simulink library "SLUGS_Library"  (Simulink 7.8)
settings: Solver=ode45  SolverMode=SingleTasking  StartTime=0.0  StopTime=10.0  RelTol=1e-3
values from neighbouring files (symbols this model uses):
  apSampleTime = 0.01    [mcuInit.m]
  derivativesConstant = 5    [mcuInit.m]
  latlong_WP = 1    [mcuInit.m]
  T = 0.01    [mcuInit.m]
  Xpoints = [0 0]    [mcuInit.m]
  Ypoints = [0 0]    [mcuInit.m]
  Zpoints = [0 0]    [mcuInit.m]
undefined symbols (not defined in the file or in its folder): bankCommandLimit, barAdjust, baroCutTemp, baroOffset, baroScale, barTGain1, barTGain2, barTMean1, barTMean2, baseHeight, baseTemp, daLimit, deLimit, DiscIntNeverNeededParam, drLimit, dtLimit, gaind, getGSLocation, getWP, GS_location, Init_onlyOnce, Init_Reset, IPStar, ISA_g, lapseRate, mass, maxAcc, MaxDwnPthStar, maxDynPressure, maxEta, Ndelay, param, pitAdjust, pitchCommandLimit, pitCutTemp, pitotOffset, pitotScale, pitTGain1, pitTGain2, pitTMean1, pitTMean2, polesd, pressureSensorCutoff, rollControlLimit, SampleT, setDiagnosticFloat, setDiagnosticShort, setLogFloat1, setLogFloat2, setNavLong, setNavNav, tanIntercept, Ts, u1, y1, yawDamperLimit, yo, zerosd
libraries: SLUGS_Library x90, simulink x37, dsPICdrivers x33, aerolibconvert2 x4, aerolibutil x1, aerolibobsolete x1
(part 6 of 7)

== system SLUGS_Library/Control Blocks/Control Blocks Examples/PID Controller w/Anti-Windup/Trapezoidal Integrator/Protect NaNs  ==
  In1 : Inport
  Integer Delay3 : Delay  DelayLength=1  InputProcessing=Inherited  SampleTime=T
  Relational Operator2 : RelationalOperator  Operator===  OutDataTypeStr=uint(8)
  Switch3 : Switch  Criteria=u2 > Threshold  Threshold=0.3  SampleTime=.01
  Out1 : Outport
  wires:
  Integer Delay3/1 -> Switch3/3
  Switch3/1 -> Out1/1, Integer Delay3/1
  In1/1 -> Relational Operator2/2, Relational Operator2/1, Switch3/1
  Relational Operator2/1 -> Switch3/2

== system SLUGS_Library/Control Blocks/Control Blocks Examples/PID Controller w/Anti-Windup/Trapezoidal Integrator/Protect NaNs1 ==
  In1 : Inport
  Integer Delay3 : Delay  DelayLength=1  InputProcessing=Inherited  SampleTime=T
  Relational Operator2 : RelationalOperator  Operator===  OutDataTypeStr=uint(8)
  Switch3 : Switch  Criteria=u2 > Threshold  Threshold=0.3  SampleTime=.01
  Out1 : Outport
  wires:
  Integer Delay3/1 -> Switch3/3
  Switch3/1 -> Out1/1, Integer Delay3/1
  In1/1 -> Relational Operator2/2, Relational Operator2/1, Switch3/1
  Relational Operator2/1 -> Switch3/2

== system SLUGS_Library/Control Blocks/Lateral Channel/Roll Control [PID]/Trapezoidal Integrator/Protect NaNs  ==
  In1 : Inport
  Integer Delay3 : Delay  DelayLength=1  InputProcessing=Inherited  SampleTime=T
  Relational Operator2 : RelationalOperator  Operator===  OutDataTypeStr=uint(8)
  Switch3 : Switch  Criteria=u2 > Threshold  Threshold=0.3  SampleTime=.01
  Out1 : Outport
  wires:
  Relational Operator2/1 -> Switch3/2
  In1/1 -> Switch3/1, Relational Operator2/1, Relational Operator2/2
  Switch3/1 -> Integer Delay3/1, Out1/1
  Integer Delay3/1 -> Switch3/3

== system SLUGS_Library/Control Blocks/Lateral Channel/Roll Control [PID]/Trapezoidal Integrator/Protect NaNs1 ==
  In1 : Inport
  Integer Delay3 : Delay  DelayLength=1  InputProcessing=Inherited  SampleTime=T
  Relational Operator2 : RelationalOperator  Operator===  OutDataTypeStr=uint(8)
  Switch3 : Switch  Criteria=u2 > Threshold  Threshold=0.3  SampleTime=.01
  Out1 : Outport
  wires:
  Relational Operator2/1 -> Switch3/2
  In1/1 -> Switch3/1, Relational Operator2/1, Relational Operator2/2
  Switch3/1 -> Integer Delay3/1, Out1/1
  Integer Delay3/1 -> Switch3/3

== system SLUGS_Library/Control Blocks/Lateral Channel/Sideslip Compensation/Low Pass/Compute Coef ==
  a : Inport
  Enable : EnablePort
  -T : Gain  Gain=-apSampleTime  SampleTime=apSampleTime
  1-c : Sum  Inputs=-+  OutDataTypeStr=single  SampleTime=apSampleTime
  Constant : Constant
  Math Function : Math  SaturateOnIntegerOverflow=on
  b : Outport
  c : Outport  Port=2
  wires:
  a/1 -> -T/1
  1-c/1 -> b/1
  Constant/1 -> 1-c/2
  Math Function/1 -> c/1, 1-c/1  "c"
  -T/1 -> Math Function/1

== system SLUGS_Library/Control Blocks/Lateral Channel/Sideslip Compensation/Low Pass/Detect Change ==
  Data : Inport
  Abs1 : Abs  SampleTime=apSampleTime
  Difference1 : simulink/Discrete/Difference  ICPrevInput=0.0  InputProcessing=Inherited  OutMin=[]  OutMax=[]  OutDataType=sfix(16)  OutScaling=2^-10  DoSatur=off
  Saturation1 : Saturate  UpperLimit=1  LowerLimit=0  SampleTime=apSampleTime
  change? : Outport
  wires:
  Saturation1/1 -> change?/1
  Data/1 -> Difference1/1
  Abs1/1 -> Saturation1/1
  Difference1/1 -> Abs1/1

== system SLUGS_Library/Control Blocks/Lateral Channel/Yaw Damper [PID]/Trapezoidal Integrator/Protect NaNs  ==
  In1 : Inport
  Integer Delay3 : Delay  DelayLength=1  InputProcessing=Inherited  SampleTime=T
  Relational Operator2 : RelationalOperator  Operator===  OutDataTypeStr=uint(8)
  Switch3 : Switch  Criteria=u2 > Threshold  Threshold=0.3  SampleTime=.01
  Out1 : Outport
  wires:
  Relational Operator2/1 -> Switch3/2
  In1/1 -> Switch3/1, Relational Operator2/1, Relational Operator2/2
  Switch3/1 -> Integer Delay3/1, Out1/1
  Integer Delay3/1 -> Switch3/3

== system SLUGS_Library/Control Blocks/Lateral Channel/Yaw Damper [PID]/Trapezoidal Integrator/Protect NaNs1 ==
  In1 : Inport
  Integer Delay3 : Delay  DelayLength=1  InputProcessing=Inherited  SampleTime=T
  Relational Operator2 : RelationalOperator  Operator===  OutDataTypeStr=uint(8)
  Switch3 : Switch  Criteria=u2 > Threshold  Threshold=0.3  SampleTime=.01
  Out1 : Outport
  wires:
  Relational Operator2/1 -> Switch3/2
  In1/1 -> Switch3/1, Relational Operator2/1, Relational Operator2/2
  Switch3/1 -> Integer Delay3/1, Out1/1
  Integer Delay3/1 -> Switch3/3

== system SLUGS_Library/Control Blocks/Longitudinal Channel/Airspeed Hold [PID]/Trapezoidal Integrator/Protect NaNs  ==
  In1 : Inport
  Integer Delay3 : Delay  DelayLength=1  InputProcessing=Inherited  SampleTime=T
  Relational Operator2 : RelationalOperator  Operator===  OutDataTypeStr=uint(8)
  Switch3 : Switch  Criteria=u2 > Threshold  Threshold=0.3  SampleTime=.01
  Out1 : Outport
  wires:
  Relational Operator2/1 -> Switch3/2
  In1/1 -> Switch3/1, Relational Operator2/1, Relational Operator2/2
  Switch3/1 -> Integer Delay3/1, Out1/1
  Integer Delay3/1 -> Switch3/3

== system SLUGS_Library/Control Blocks/Longitudinal Channel/Airspeed Hold [PID]/Trapezoidal Integrator/Protect NaNs1 ==
  In1 : Inport
  Integer Delay3 : Delay  DelayLength=1  InputProcessing=Inherited  SampleTime=T
  Relational Operator2 : RelationalOperator  Operator===  OutDataTypeStr=uint(8)
  Switch3 : Switch  Criteria=u2 > Threshold  Threshold=0.3  SampleTime=.01
  Out1 : Outport
  wires:
  Relational Operator2/1 -> Switch3/2
  In1/1 -> Switch3/1, Relational Operator2/1, Relational Operator2/2
  Switch3/1 -> Integer Delay3/1, Out1/1
  Integer Delay3/1 -> Switch3/3

== system SLUGS_Library/Control Blocks/Longitudinal Channel/Height Error to Pitch  Command [PI]/Trapezoidal Integrator/Protect NaNs ==
  In1 : Inport
  Integer Delay3 : Delay  DelayLength=1  InputProcessing=Inherited  SampleTime=T
  Relational Operator2 : RelationalOperator  Operator===  OutDataTypeStr=uint(8)
  Switch3 : Switch  Criteria=u2 > Threshold  Threshold=0.3  SampleTime=.01
  Out1 : Outport
  wires:
  Relational Operator2/1 -> Switch3/2
  In1/1 -> Switch3/1, Relational Operator2/1, Relational Operator2/2
  Switch3/1 -> Integer Delay3/1, Out1/1
  Integer Delay3/1 -> Switch3/3

== system SLUGS_Library/Control Blocks/Longitudinal Channel/Height Error to Pitch  Command [PI]/Trapezoidal Integrator/Protect NaNs  ==
  In1 : Inport
  Integer Delay3 : Delay  DelayLength=1  InputProcessing=Inherited  SampleTime=T
  Relational Operator2 : RelationalOperator  Operator===  OutDataTypeStr=uint(8)
  Switch3 : Switch  Criteria=u2 > Threshold  Threshold=0.3  SampleTime=.01
  Out1 : Outport
  wires:
  Relational Operator2/1 -> Switch3/2
  In1/1 -> Switch3/1, Relational Operator2/1, Relational Operator2/2
  Switch3/1 -> Integer Delay3/1, Out1/1
  Integer Delay3/1 -> Switch3/3

== system SLUGS_Library/Control Blocks/Longitudinal Channel/Pitch To Elevator [PID]/Trapezoidal Integrator/Protect NaNs  ==
  In1 : Inport
  Integer Delay3 : Delay  DelayLength=1  InputProcessing=Inherited  SampleTime=T
  Relational Operator2 : RelationalOperator  Operator===  OutDataTypeStr=uint(8)
  Switch3 : Switch  Criteria=u2 > Threshold  Threshold=0.3  SampleTime=.01
  Out1 : Outport
  wires:
  Relational Operator2/1 -> Switch3/2
  In1/1 -> Switch3/1, Relational Operator2/1, Relational Operator2/2
  Switch3/1 -> Integer Delay3/1, Out1/1
  Integer Delay3/1 -> Switch3/3

== system SLUGS_Library/Control Blocks/Longitudinal Channel/Pitch To Elevator [PID]/Trapezoidal Integrator/Protect NaNs1 ==
  In1 : Inport
  Integer Delay3 : Delay  DelayLength=1  InputProcessing=Inherited  SampleTime=T
  Relational Operator2 : RelationalOperator  Operator===  OutDataTypeStr=uint(8)
  Switch3 : Switch  Criteria=u2 > Threshold  Threshold=0.3  SampleTime=.01
  Out1 : Outport
  wires:
  Relational Operator2/1 -> Switch3/2
  In1/1 -> Switch3/1, Relational Operator2/1, Relational Operator2/2
  Switch3/1 -> Integer Delay3/1, Out1/1
  Integer Delay3/1 -> Switch3/3

== system SLUGS_Library/InnerLoop/Longitudinal Channel/Airspeed Hold [PID]/Trapezoidal Integrator/Protect NaNs  ==
  In1 : Inport
  Integer Delay3 : Delay  DelayLength=1  InputProcessing=Inherited  SampleTime=T
  Relational Operator2 : RelationalOperator  Operator===  OutDataTypeStr=uint(8)
  Switch3 : Switch  Criteria=u2 > Threshold  Threshold=0.3  SampleTime=.01
  Out1 : Outport
  wires:
  Integer Delay3/1 -> Switch3/3
  Switch3/1 -> Out1/1, Integer Delay3/1
  In1/1 -> Relational Operator2/2, Relational Operator2/1, Switch3/1
  Relational Operator2/1 -> Switch3/2

== system SLUGS_Library/InnerLoop/Longitudinal Channel/Airspeed Hold [PID]/Trapezoidal Integrator/Protect NaNs1 ==
  In1 : Inport
  Integer Delay3 : Delay  DelayLength=1  InputProcessing=Inherited  SampleTime=T
  Relational Operator2 : RelationalOperator  Operator===  OutDataTypeStr=uint(8)
  Switch3 : Switch  Criteria=u2 > Threshold  Threshold=0.3  SampleTime=.01
  Out1 : Outport
  wires:
  Integer Delay3/1 -> Switch3/3
  Switch3/1 -> Out1/1, Integer Delay3/1
  In1/1 -> Relational Operator2/2, Relational Operator2/1, Switch3/1
  Relational Operator2/1 -> Switch3/2

== system SLUGS_Library/InnerLoop/Longitudinal Channel/Height Error to Pitch  Command [PI]/Trapezoidal Integrator/Protect NaNs ==
  In1 : Inport
  Integer Delay3 : Delay  DelayLength=1  InputProcessing=Inherited  SampleTime=T
  Relational Operator2 : RelationalOperator  Operator===  OutDataTypeStr=uint(8)
  Switch3 : Switch  Criteria=u2 > Threshold  Threshold=0.3  SampleTime=.01
  Out1 : Outport
  wires:
  Integer Delay3/1 -> Switch3/3
  Switch3/1 -> Out1/1, Integer Delay3/1
  In1/1 -> Relational Operator2/2, Relational Operator2/1, Switch3/1
  Relational Operator2/1 -> Switch3/2

== system SLUGS_Library/InnerLoop/Longitudinal Channel/Height Error to Pitch  Command [PI]/Trapezoidal Integrator/Protect NaNs  ==
  In1 : Inport
  Integer Delay3 : Delay  DelayLength=1  InputProcessing=Inherited  SampleTime=T
  Relational Operator2 : RelationalOperator  Operator===  OutDataTypeStr=uint(8)
  Switch3 : Switch  Criteria=u2 > Threshold  Threshold=0.3  SampleTime=.01
  Out1 : Outport
  wires:
  Integer Delay3/1 -> Switch3/3
  Switch3/1 -> Out1/1, Integer Delay3/1
  In1/1 -> Relational Operator2/2, Relational Operator2/1, Switch3/1
  Relational Operator2/1 -> Switch3/2

== system SLUGS_Library/InnerLoop/Longitudinal Channel/Pitch To Elevator [PID]/Trapezoidal Integrator/Protect NaNs  ==
  In1 : Inport
  Integer Delay3 : Delay  DelayLength=1  InputProcessing=Inherited  SampleTime=T
  Relational Operator2 : RelationalOperator  Operator===  OutDataTypeStr=uint(8)
  Switch3 : Switch  Criteria=u2 > Threshold  Threshold=0.3  SampleTime=.01
  Out1 : Outport
  wires:
  Integer Delay3/1 -> Switch3/3
  Switch3/1 -> Out1/1, Integer Delay3/1
  In1/1 -> Relational Operator2/2, Relational Operator2/1, Switch3/1
  Relational Operator2/1 -> Switch3/2

== system SLUGS_Library/InnerLoop/Longitudinal Channel/Pitch To Elevator [PID]/Trapezoidal Integrator/Protect NaNs1 ==
  In1 : Inport
  Integer Delay3 : Delay  DelayLength=1  InputProcessing=Inherited  SampleTime=T
  Relational Operator2 : RelationalOperator  Operator===  OutDataTypeStr=uint(8)
  Switch3 : Switch  Criteria=u2 > Threshold  Threshold=0.3  SampleTime=.01
  Out1 : Outport
  wires:
  Integer Delay3/1 -> Switch3/3
  Switch3/1 -> Out1/1, Integer Delay3/1
  In1/1 -> Relational Operator2/2, Relational Operator2/1, Switch3/1
  Relational Operator2/1 -> Switch3/2

== system SLUGS_Library/InnerLoop/Navigation/Compute WP Index/Compute Modified L1/Compute T  in Frenet ==
  Pos 1 : Inport
  Pos 2 : Inport  Port=2
  Add : Sum  Inputs=-+
  Normalize Vector : SLUGS_Library/Navigation/Normalize Vector
  T : Outport
  wires:
  Pos 1/1 -> Add/1
  Pos 2/1 -> Add/2
  Add/1 -> Normalize Vector/1
  Normalize Vector/1 -> T/1

== system SLUGS_Library/InnerLoop/Navigation/Compute WP Index/Compute Modified L1/Get Circles ==
  T1 : Inport
  T2 : Inport  Port=2
  "Wp_to " : Inport  Port=3
  R : Inport  Port=4
  Compute  Circles : MATLAB Function  TreatAsAtomicUnit=on
  Compute CCW Angle From 2 Vectors : Subsystem
  Compute delta Left Turn : Subsystem
  Constant5 : Constant  Value=pi  OutDataTypeStr=single
  Larger than 180? : RelationalOperator  OutDataTypeStr=boolean
  Logical Operator : Logic  Operator=NOT  AllPortsSameDT=off  OutDataTypeStr=boolean
  Merge4 : Merge
  Subsystem5 : SLUGS_Library/Subsystem5
  To Workspace : ToWorkspace  VariableName=O  SampleTime=-1  SaveFormat=Structure
  To Workspace1 : ToWorkspace  VariableName=P  SampleTime=-1  SaveFormat=Structure
  To Workspace2 : ToWorkspace  VariableName=Pch  SampleTime=-1  SaveFormat=Structure
  To Workspace3 : ToWorkspace  VariableName=PchB  SampleTime=-1  SaveFormat=Structure
  compute delta Right Turn : Subsystem
  P : Outport
  wires:
  Subsystem5/2 -> Compute  Circles/2(cd)
  Subsystem5/1 -> Compute  Circles/1(sd)
  Logical Operator/1 -> Compute delta Left Turn/Enable
  Larger than 180?/1 -> Logical Operator/1, compute delta Right Turn/Enable
  Constant5/1 -> Larger than 180?/2
  Compute  Circles/4(PchB) -> To Workspace3/1
  Compute  Circles/3(Pch) -> To Workspace2/1
  Compute  Circles/2(P) -> To Workspace1/1, P/1
  Compute  Circles/1(O) -> To Workspace/1
  "Wp_to "/1 -> Compute  Circles/3(WP1)
  R/1 -> Compute  Circles/4(R)
  Compute delta Left Turn/1(delta) -> Merge4/2
  compute delta Right Turn/1(delta) -> Merge4/1
  Merge4/1 -> Subsystem5/1
  T2/1 -> Compute CCW Angle From 2 Vectors/2(V), Compute  Circles/6(T2)
  Compute CCW Angle From 2 Vectors/1(CCW Ang) -> Larger than 180?/1, compute delta Right Turn/1(gamma), Compute delta Left Turn/1(gamma)  "gamma"
  T1/1 -> Compute CCW Angle From 2 Vectors/1(U), Compute  Circles/5(T1)

== system SLUGS_Library/InnerLoop/Navigation/Compute WP Index/Compute Modified L1/get WP Coord from Index ==
  WP Idx : Inport
  C Function Call : dsPICdrivers/OTHERS/C Function Call  Tag=dsPIC_dsPIC_CFunctionCall  FctUpdate=Output Function  fctName='getWP'  INPUT_SIZE=1  INPUT1=uint8  INPUT2=--  INPUT3=--  OUTPUT_SIZE=3  OUTPUT1=real32  SampleTime=-1  InputType=[ 2 ]  OutputType=[ 7 ]  FctDeclaration=extern void getWP(uint8_T u1,real32_T* y1);  FctCall=getWP(%u1, *%y1);  OrderingInOutPopup=None  FctStart=None  FctStart_Name=Init_onlyOnce  FctStart_Declaration=inline extern void Init_onlyOnce();  FctStart_Call=Init_onlyOnce();  FctInit=None  FctInit_Name=Init_Reset  FctInit_Declaration=inline extern void Init_Reset();  FctInit_Call=Init_Reset();  PinDigitalInput=[]  PinDigitalOutput=[]  AnalogueInput=[]
  Data Type Conversion : DataTypeConversion  OutDataTypeStr=double
  Data Type Conversion1 : DataTypeConversion  OutDataTypeStr=single
  Environment Controller : simulink/Signal Routing/Environment Controller
  MATLAB Fcn : MATLABFcn  MATLABFcn=Xpoints(u(1))  OutputDimensions=1  OutputSignalType=real
  MATLAB Fcn1 : MATLABFcn  MATLABFcn=Ypoints(u(1))  OutputDimensions=1
  MATLAB Fcn2 : MATLABFcn  MATLABFcn=Zpoints(u(1))  OutputDimensions=1
  Mux : Mux  Inputs=3
  WP Coord : Outport
  wires:
  C Function Call/1 -> Environment Controller/2
  Environment Controller/1 -> WP Coord/1
  Mux/1 -> Data Type Conversion1/1
  WP Idx/1 -> C Function Call/1, Data Type Conversion/1
  MATLAB Fcn2/1 -> Mux/3
  MATLAB Fcn1/1 -> Mux/2
  MATLAB Fcn/1 -> Mux/1
  Data Type Conversion/1 -> MATLAB Fcn1/1, MATLAB Fcn/1, MATLAB Fcn2/1
  Data Type Conversion1/1 -> Environment Controller/1

== system SLUGS_Library/Navigation/Compute WP Index/Compute Modified L1/Get Circles/Compute CCW Angle From 2 Vectors ==
  U : Inport
  V : Inport  Port=2
  Add : Sum  Inputs=+-
  Embedded MATLAB Function1 : MATLAB Function  TreatAsAtomicUnit=on
  Selector : Selector  InputPortWidth=3  IndexOptions=Index vector (dialog)  Indices=[1]  OutputSizes=1
  Selector1 : Selector  InputPortWidth=3  IndexOptions=Index vector (dialog)  Indices=[1]  OutputSizes=1
  Selector2 : Selector  InputPortWidth=3  IndexOptions=Index vector (dialog)  Indices=[2]  OutputSizes=1
  Selector3 : Selector  InputPortWidth=3  IndexOptions=Index vector (dialog)  Indices=[2]  OutputSizes=1
  Subsystem1 : SLUGS_Library/Subsystem4
  Subsystem4 : SLUGS_Library/Subsystem4
  CCW Ang : Outport
  wires:
  Selector3/1 -> Subsystem4/1
  Selector/1 -> Subsystem4/2
  Selector2/1 -> Subsystem1/1
  Selector1/1 -> Subsystem1/2
  Subsystem4/1 -> Add/1
  Subsystem1/1 -> Add/2
  Add/1 -> Embedded MATLAB Function1/1(rawAngle)
  U/1 -> Selector3/1, Selector/1
  V/1 -> Selector2/1, Selector1/1
  Embedded MATLAB Function1/1(angle) -> CCW Ang/1

== system SLUGS_Library/Navigation/Compute WP Index/Compute Modified L1/Get Circles/Compute delta Left Turn ==
  gamma : Inport
  Enable : EnablePort
  Add : Sum  Inputs=+-
  Constant1 : Constant  Value=2
  Constant5 : Constant  Value=pi
  Divide : Product  Inputs=*/
  Gain : Gain  Gain=-1
  delta : Outport
  wires:
  Constant1/1 -> Divide/2
  Divide/1 -> Gain/1
  Constant5/1 -> Add/1
  gamma/1 -> Add/2
  Add/1 -> Divide/1
  Gain/1 -> delta/1

== system SLUGS_Library/Navigation/Compute WP Index/Compute Modified L1/Get Circles/compute delta Right Turn ==
  gamma : Inport
  Enable : EnablePort
  Add : Sum  Inputs=-+
  Constant1 : Constant  Value=2
  Constant5 : Constant  Value=pi
  Divide : Product  Inputs=*/
  delta : Outport
  wires:
  Constant5/1 -> Add/1
  Add/1 -> Divide/1
  Constant1/1 -> Divide/2
  gamma/1 -> Add/2
  Divide/1 -> delta/1  "delta"

== system SLUGS_Library/Navigation/Geod2LTP/ECEF2LTP (UEN)/From Body to Universal1/Rotation Matrix from Long//Lat ==
  note: Calculate Coefficients of DCM Row-Wise
  long lat : Inport
  11 : Fcn  Expr=cos(u[1])*cos(u[2])
  12 : Fcn  Expr=sin(u[1])*cos(u[2])
  13 : Fcn  Expr=sin(u[2])
  21 : Fcn  Expr=-sin(u[1])
  22 : Fcn  Expr=cos(u[1])
  23 : Fcn  Expr=0
  31 : Fcn  Expr=-sin(u[2])*cos(u[1])
  32 : Fcn  Expr=-sin(u[1])*sin(u[2])
  33 : Fcn  Expr=cos(u[2])
  Mux2 : Mux  Inputs=9
  DCM : Outport
  wires:
  long lat/1 -> 21/1, 31/1, 12/1, 22/1, 32/1, 13/1, 23/1, 33/1, 11/1
  Mux2/1 -> DCM/1
  11/1 -> Mux2/1
  21/1 -> Mux2/2
  31/1 -> Mux2/3
  12/1 -> Mux2/4
  22/1 -> Mux2/5
  32/1 -> Mux2/6
  13/1 -> Mux2/7
  23/1 -> Mux2/8
  33/1 -> Mux2/9

== system SLUGS_Library/Navigation/Navigation/L2+/Get Sin, Cos eta/2D Dot Product  ==
  Vxyz : Inport
  L2_vec : Inport  Port=2
  Demux : Demux  Outputs=3
  Demux1 : Demux  Outputs=3
  Product : Product  RndMeth=Zero
  Product1 : Product  RndMeth=Zero
  Subtract : Sum  Inputs=2
  Terminator : Terminator
  Terminator1 : Terminator
  2D _dot : Outport
  wires:
  Vxyz/1 -> Demux/1
  Subtract/1 -> 2D _dot/1
  L2_vec/1 -> Demux1/1
  Product1/1 -> Subtract/2
  Product/1 -> Subtract/1
  Demux1/3 -> Terminator1/1
  Demux/3 -> Terminator/1
  Demux1/1 -> Product/1
  Demux/1 -> Product/2
  Demux1/2 -> Product1/1
  Demux/2 -> Product1/2

== system SLUGS_Library/Navigation/Navigation/L2+/Get Sin, Cos eta/Get  Groundspeed ==
  L2_vec : Inport  SampleTime=apSampleTime
  Vector Norm : SLUGS_Library/Vector Norm
  Zero out Z1 : MATLAB Function  TreatAsAtomicUnit=on
  |L2| : Outport
  wires:
  L2_vec/1 -> Zero out Z1/1(Pin)
  Zero out Z1/1(P) -> Vector Norm/1
  Vector Norm/1 -> |L2|/1

== system SLUGS_Library/Navigation/Navigation/L2+/Get Sin, Cos eta/Get ZProd ==
  L2_vec : Inport
  Vxyz : Inport  Port=2
  Demux : Demux  Outputs=3
  Demux1 : Demux  Outputs=3
  Product : Product  RndMeth=Zero
  Product1 : Product  RndMeth=Zero
  Subtract : Sum  Inputs=+-
  Terminator : Terminator
  Terminator1 : Terminator
  Z_prod : Outport
  wires:
  Demux/3 -> Terminator/1
  Demux1/3 -> Terminator1/1
  Demux/1 -> Product/2
  Demux1/2 -> Product/1
  Demux/2 -> Product1/2
  Demux1/1 -> Product1/1
  Product/1 -> Subtract/1
  Product1/1 -> Subtract/2
  L2_vec/1 -> Demux1/1
  Subtract/1 -> Z_prod/1
  Vxyz/1 -> Demux/1

== system SLUGS_Library/Navigation/Navigation/Normal WP  Navigation/Compute WP Switching Trigger/Compute  Projection ==
  Pned : Inport
  ToWp : Inport  Port=2
  T : Inport  Port=3
  Protect NaNs : Subsystem
  Subtract : Sum  Inputs=-+  OutDataTypeStr=single
  dsPIC Dot Product : SLUGS_Library/dsPIC Dot Product
  D2wp1 : Outport
  wires:
  Protect NaNs/1(Out1) -> D2wp1/1
  Pned/1 -> Subtract/1
  ToWp/1 -> Subtract/2
  Subtract/1 -> dsPIC Dot Product/1
  T/1 -> dsPIC Dot Product/2
  dsPIC Dot Product/1 -> Protect NaNs/1(In1)

== system SLUGS_Library/Navigation/Navigation/Normal WP  Navigation/On WP Enable/Subsystem ==
  GS LLA : Inport
  GS R_in : Inport  Port=2
  Compute Frenet : SLUGS_Library/Navigation/Compute Frenet
  Constant : Constant  OutDataTypeStr=uint8  SampleTime=0.01
  Constant1 : Constant  Value=2  OutDataTypeStr=uint8  SampleTime=0.01
  GS LLA_1 : InportShadow  Port=1
  GS R_in_1 : InportShadow  Port=2
  Terminator : Terminator
  get WP Coord from Index : SLUGS_Library/Navigation/get WP Coord from Index
  get WP Coord from Index1 : SLUGS_Library/Navigation/get WP Coord from Index
  WP0 : Outport
  T1 : Outport  Port=2
  wires:
  GS R_in_1/1 -> get WP Coord from Index1/3
  GS LLA_1/1 -> get WP Coord from Index1/2
  Constant1/1 -> get WP Coord from Index1/1
  get WP Coord from Index1/1 -> Compute Frenet/2
  get WP Coord from Index/1 -> Compute Frenet/1, WP0/1
  GS R_in/1 -> get WP Coord from Index/3
  GS LLA/1 -> get WP Coord from Index/2
  Compute Frenet/1 -> T1/1
  Compute Frenet/2 -> Terminator/1
  Constant/1 -> get WP Coord from Index/1

== system SLUGS_Library/Navigation/Navigation/Recent Enable/Grab Upon Enable/Compute GS Location ==
  GS Location : Inport
  Demux : Demux  Outputs=3
  Geod2ECEF1 : Subsystem  mask{Re=6378137, Rp=6356752.3142}
      mask prompts: Re "Enter equatorial radius, m"; Rp "Enter polar radius,m"
  Mux1 : Mux  Inputs=2
  Mux2 : Mux  Inputs=3
  "Lon, Lat" : Outport
  R_in : Outport  Port=2
  wires:
  Geod2ECEF1/3("Ze, m ") -> Mux2/3
  Geod2ECEF1/1("Xe, m ") -> Mux2/1
  Geod2ECEF1/2("Ye, m ") -> Mux2/2
  Demux/1 -> Geod2ECEF1/1("height, m")
  Demux/2 -> Geod2ECEF1/2("lat, deg"), Mux1/2
  Demux/3 -> Geod2ECEF1/3(lon,deg), Mux1/1
  GS Location/1 -> Demux/1
  Mux1/1 -> "Lon, Lat"/1
  Mux2/1 -> R_in/1  "R_in"

== system SLUGS_Library/Navigation/Navigation/Recent Enable/Subsystem/Detect Rising Edge ==
  In1 : Inport
  Delay : Delay  DelayLength=1
  Logical Operator : Logic  AllPortsSameDT=off  OutDataTypeStr=boolean
  Relational Operator : RelationalOperator  Operator=~=  OutDataTypeStr=boolean
  Out1 : Outport
  wires:
  Logical Operator/1 -> Out1/1
  In1/1 -> Logical Operator/2, Relational Operator/2, Delay/1
  Relational Operator/1 -> Logical Operator/1
  Delay/1 -> Relational Operator/1

== system SLUGS_Library/Sensor Blocks/Baro Alt/Baro Altimeter/Initial Baro Bias/Low Pass8 ==
  In1 : Inport
  Discrete Zero-Pole : DiscreteZeroPole  Zeros=zerosd  Poles=polesd  Gain=gaind  SampleTime=SampleTime
  Out1 : Outport
  wires:
  In1/1 -> Discrete Zero-Pole/1
  Discrete Zero-Pole/1 -> Out1/1

== system SLUGS_Library/InnerLoop/Navigation/Compute WP Index/Compute Modified L1/Get Circles/Compute CCW Angle From 2 Vectors ==
  U : Inport
  V : Inport  Port=2
  Add : Sum  Inputs=+-
  Embedded MATLAB Function1 : MATLAB Function  TreatAsAtomicUnit=on
  Selector : Selector  InputPortWidth=3  IndexOptions=Index vector (dialog)  Indices=[1]  OutputSizes=1
  Selector1 : Selector  InputPortWidth=3  IndexOptions=Index vector (dialog)  Indices=[1]  OutputSizes=1
  Selector2 : Selector  InputPortWidth=3  IndexOptions=Index vector (dialog)  Indices=[2]  OutputSizes=1
  Selector3 : Selector  InputPortWidth=3  IndexOptions=Index vector (dialog)  Indices=[2]  OutputSizes=1
  Subsystem1 : SLUGS_Library/Subsystem4
  Subsystem4 : SLUGS_Library/Subsystem4
  CCW Ang : Outport
  wires:
  Embedded MATLAB Function1/1(angle) -> CCW Ang/1
  V/1 -> Selector1/1, Selector2/1
  U/1 -> Selector/1, Selector3/1
  Add/1 -> Embedded MATLAB Function1/1(rawAngle)
  Subsystem1/1 -> Add/2
  Subsystem4/1 -> Add/1
  Selector1/1 -> Subsystem1/2
  Selector2/1 -> Subsystem1/1
  Selector/1 -> Subsystem4/2
  Selector3/1 -> Subsystem4/1

== system SLUGS_Library/InnerLoop/Navigation/Compute WP Index/Compute Modified L1/Get Circles/Compute delta Left Turn ==
  gamma : Inport
  Enable : EnablePort
  Add : Sum  Inputs=+-  OutDataTypeStr=single
  Constant1 : Constant  Value=2  OutDataTypeStr=single
  Constant5 : Constant  Value=pi  OutDataTypeStr=single
  Divide : Product  Inputs=*/  OutDataTypeStr=single
  Gain : Gain  Gain=-1
  delta : Outport
  wires:
  Gain/1 -> delta/1
  Add/1 -> Divide/1
  gamma/1 -> Add/2
  Constant5/1 -> Add/1
  Divide/1 -> Gain/1
  Constant1/1 -> Divide/2

== system SLUGS_Library/InnerLoop/Navigation/Compute WP Index/Compute Modified L1/Get Circles/compute delta Right Turn ==
  gamma : Inport
  Enable : EnablePort
  Add : Sum  Inputs=-+  OutDataTypeStr=single
  Constant1 : Constant  Value=2  OutDataTypeStr=single
  Constant5 : Constant  Value=pi  OutDataTypeStr=single
  Divide : Product  Inputs=*/  OutDataTypeStr=single
  delta : Outport
  wires:
  Divide/1 -> delta/1  "delta"
  gamma/1 -> Add/2
  Constant1/1 -> Divide/2
  Add/1 -> Divide/1
  Constant5/1 -> Add/1

== system SLUGS_Library/Navigation/Navigation/Normal WP  Navigation/Compute WP Switching Trigger/Compute  Projection/Protect NaNs ==
  In1 : Inport
  Integer Delay3 : Delay  DelayLength=1  InputProcessing=Inherited  SampleTime=T
  Relational Operator2 : RelationalOperator  Operator===  OutDataTypeStr=uint(8)
  Switch3 : Switch  Criteria=u2 > Threshold  Threshold=0.3  SampleTime=.01
  Out1 : Outport
  wires:
  Integer Delay3/1 -> Switch3/3
  Switch3/1 -> Out1/1, Integer Delay3/1
  In1/1 -> Relational Operator2/2, Relational Operator2/1, Switch3/1
  Relational Operator2/1 -> Switch3/2

== system SLUGS_Library/Navigation/Navigation/Recent Enable/Grab Upon Enable/Compute GS Location/Geod2ECEF1 ==
  "height, m" : Inport
  "lat, deg" : Inport  Port=2
  lon,deg : Inport  Port=3
  (Rh+h)cos(phi)*cos(lamb)=Xe : Product  Inputs=3  OutDataTypeStr=single  SaturateOnIntegerOverflow=on  InputSameDT=on
  (Rh+h)cos(phi)*sin(lamb)=Ye : Product  Inputs=3  OutDataTypeStr=single  SaturateOnIntegerOverflow=on  InputSameDT=on
  Deg2R : Gain  Gain=pi/180  OutDataTypeStr=float('single')  SaturateOnIntegerOverflow=on  ParamDataTypeStr=Inherit: Same as input
  Deg2R1 : Gain  Gain=pi/180  OutDataTypeStr=float('single')  SaturateOnIntegerOverflow=on  ParamDataTypeStr=Inherit: Same as input
  Product1 : Product  SaturateOnIntegerOverflow=on  InputSameDT=on  OutDataTypeStr=Inherit: Same as first input
  Re=equatorial radius : Constant  Value=Re  OutDataTypeStr=single
  Rh : Product  Inputs=*/  OutDataTypeStr=single  SaturateOnIntegerOverflow=on  InputSameDT=on
  Rh(1-e^2) : Product  OutDataTypeStr=single  SaturateOnIntegerOverflow=on  InputSameDT=on
  Sum1 : Sum  Inputs=+-|  SaturateOnIntegerOverflow=on  InputSameDT=on  OutDataTypeStr=Inherit: Same as first input
  Sum2 : Sum  SaturateOnIntegerOverflow=on  InputSameDT=on  OutDataTypeStr=Inherit: Same as first input
      settings: AttributesFormatString=Rh+h
  Sum3 : Sum  Inputs=|+-  SaturateOnIntegerOverflow=on  InputSameDT=on  OutDataTypeStr=Inherit: Same as first input
  Sum4 : Sum  OutDataTypeStr=single  SaturateOnIntegerOverflow=on  InputSameDT=on
      settings: AttributesFormatString=(1-e^2)Rh+h
  Ze : Product  OutDataTypeStr=single  SaturateOnIntegerOverflow=on  InputSameDT=on
  const : Constant  OutDataTypeStr=single
  const1 : Constant  OutDataTypeStr=single
  cos(lamb) : Trigonometry  Operator=cos
  cos(phi) : Trigonometry  Operator=cos
  eccentricity^2 : Subsystem
  f : Fcn  Expr=sqrt(u(1))
  sin(lamb) : Trigonometry
  sin(phi) : Trigonometry
  sin(phi)^2 : Product  SaturateOnIntegerOverflow=on  InputSameDT=on  OutDataTypeStr=Inherit: Same as first input
  "Xe, m " : Outport
  "Ye, m " : Outport  Port=2
  "Ze, m " : Outport  Port=3
  wires:
  (Rh+h)cos(phi)*sin(lamb)=Ye/1 -> "Ye, m "/1
  (Rh+h)cos(phi)*cos(lamb)=Xe/1 -> "Xe, m "/1
  Sum2/1 -> (Rh+h)cos(phi)*cos(lamb)=Xe/1, (Rh+h)cos(phi)*sin(lamb)=Ye/1
  Deg2R1/1 -> sin(lamb)/1, cos(lamb)/1
  Deg2R/1 -> sin(phi)/1, cos(phi)/1
  Ze/1 -> "Ze, m "/1
  sin(lamb)/1 -> (Rh+h)cos(phi)*sin(lamb)=Ye/3
  cos(lamb)/1 -> (Rh+h)cos(phi)*cos(lamb)=Xe/3
  cos(phi)/1 -> (Rh+h)cos(phi)*sin(lamb)=Ye/2, (Rh+h)cos(phi)*cos(lamb)=Xe/2
  lon,deg/1 -> Deg2R1/1
  Sum4/1 -> Ze/2
  Rh(1-e^2)/1 -> Sum4/1
  Sum3/1 -> Rh(1-e^2)/1  "1-e^2"
  const1/1 -> Sum3/1
  sin(phi)^2/1 -> Product1/2
  eccentricity^2/1(e^2) -> Sum3/2, Product1/1
  "height, m"/1 -> Sum2/1, Sum4/2
  const/1 -> Sum1/1
  Sum1/1 -> f/1
  Product1/1 -> Sum1/2
  Rh/1 -> Rh(1-e^2)/2, Sum2/2
  Re=equatorial radius/1 -> Rh/1
  f/1 -> Rh/2
  sin(phi)/1 -> Ze/1, sin(phi)^2/2, sin(phi)^2/1
  "lat, deg"/1 -> Deg2R/1

== system SLUGS_Library/Navigation/Navigation/Recent Enable/Grab Upon Enable/Compute GS Location/Geod2ECEF1/eccentricity^2 ==
  " " : Product  OutDataTypeStr=single  SaturateOnIntegerOverflow=on  InputSameDT=on
  Re=equatorial radius1 : Constant  Value=Re  OutDataTypeStr=single
  Rp=polar radius : Constant  Value=Rp  OutDataTypeStr=single
  Sum5 : Sum  Inputs=|+-  SaturateOnIntegerOverflow=on  InputSameDT=on  OutDataTypeStr=Inherit: Same as first input
  const2 : Constant  OutDataTypeStr=single
  e^1 : Product  Inputs=*/  OutDataTypeStr=single  SaturateOnIntegerOverflow=on  InputSameDT=on
  e^2 : Outport
  wires:
  Sum5/1 -> e^2/1
  " "/1 -> Sum5/2
  e^1/1 -> " "/1, " "/2
  const2/1 -> Sum5/1
  Rp=polar radius/1 -> e^1/1
  Re=equatorial radius1/1 -> e^1/2

== matlab function Singnal Routing & Conditioning/3D Filter/myMux Fun1 ==
  data: u1 input double; y output double; u2 input double; u3 input double
function y = myMux(u1, u2, u3)
% This block supports an embeddable subset of the MATLAB language.
% See the help menu for details. 

y = [u1(1); u2(1); u3(1)];

== matlab function Navigation/Compute Frenet/Select N Terms ==
  data: T input double; N output double
function N = getN(T)
% This block supports an embeddable subset of the MATLAB language.
% See the help menu for details. 

N = [-T(2); T(1); 0];

== matlab function Navigation/Compute WP Index/Compute Modified L1/Get Circles/Compute CCW Angle From 2 Vectors/Embedded MATLAB Function1 ==
  data: rawAngle input double; angle output double
function angle = mapToTwoPi(rawAngle)

 if(rawAngle < 0)
  angle = rawAngle + 2*pi;
 else
  angle = rawAngle;   
 end

== matlab function Compute CCW Angle From 2 Vectors/Embedded MATLAB Function1 ==
  data: rawAngle input double; angle output double
function angle = mapToTwoPi(rawAngle)

angle = rawAngle;

 if(angle < 0)
     while (angle <0)
        angle = angle + 2*pi;
     end;
 else
     while (angle > 2*pi)
        angle = angle - 2*pi;
     end
 end

== matlab function dsPIC Dot Product/Embedded MATLAB Function ==
  data: x input double; y input double; xDoty output double
function xDoty = myDot(x,y)
% This block supports an embeddable subset of the MATLAB language.
% See the help menu for details. 

xDoty = x(1)*y(1) + x(2)*y(2) + x(3)*y(3);

== matlab function Embedded MATLAB Function ==
  data: T1 input double; gamma output double; T2 input double
function gamma = computeAngle(T1, T2)
% This block supports an embeddable subset of the MATLAB language.
% See the help menu for details. 

gamma = (atan2(T1(2), T1(1)) - atan2(T2(2), T2(1)));

 if(gamma < 0)
  gamma = gamma + 2*pi;
 end

== matlab function Navigation/Compute WP Index/Embedded MATLAB Function ==
  data: wpStart input double; wpCount input double; wp0 output double; swIncrement input double; wp1 output double; wp2 output double; wpEnabl input double
function [wp0,wp1, wp2] = getNextWP(wpStart, wpCount, swIncrement, wpEnabl)

% Declare static variables
persistent fromWP;
persistent toWP;
persistent totoWP;

%initialize the static variables
if isempty(fromWP)
    fromWP = wpStart;
    toWP = fromWP+1;
    % check if there are more than 2 WPs
    if wpCount > toWP + 1
        totoWP = toWP+1;
    else
        totoWP = fromWP;
    end
end

%if WP Nav was just enabled
if wpEnabl == 1
    fromWP =0;
    toWP =1;
    totoWP = 2;
end;

% if there is a change of wp
if swIncrement == 1
    fromWP = toWP;
    toWP = totoWP;
    totoWP = totoWP +1;
    if (totoWP>wpCount)
        totoWP = wpStart;
    end
end

wp0 = fromWP;
wp1 = toWP;
wp2 = totoWP;

== matlab function InnerLoop/Navigation/Compute WP Index/Compute Modified L1/Get Circles/Compute Circles ==
  data: sd input double; O output double; cd input double; WP1 input double; R input double; T1 input double; P output double; Pch output double; T2 input double; PchB output double
function [O,P,Pch, PchB] = getO(sd, cd, WP1, R, T1, T2)
    % This block supports an embeddable subset of the MATLAB language.
    % See the help menu for details.

    % rotate the vector delta degrees
    r_vec = zeros(3,1);
    r_vec(1) = -T1(1)*cd -T1(2)*sd;
    r_vec(2) = T1(1)*sd -T1(2)*cd;

    %compute M
    if localAbs(sd)>0.01
        M = localAbs(R/sd);
    else
        M = single(0);
    end

    %find the distance from WP
    P = M*cd;

    % find the center of the circle
    O = WP1 + r_vec.*M;

    % find the tangent points
    Pch = WP1-T1*P;
    PchB = WP1 + T2*P;
end

function absVal = localAbs(x)
    if x < 0
        absVal = single(-1*x);
    else
        absVal = single(x);
    end
end

== matlab function InnerLoop/Navigation/Compute WP Index/Compute Modified L1/Get Circles/Compute CCW Angle From 2 Vectors/Embedded MATLAB Function1 ==
  data: rawAngle input double; angle output double
function angle = mapToTwoPi(rawAngle)

 if(rawAngle < 0)
  angle = rawAngle + 2*pi;
 else
  angle = rawAngle;   
 end

== matlab function InnerLoop/Navigation/Compute WP Index/Embedded MATLAB Function ==
  data: wpStart input double; wpCount input double; wp0 output double; swIncrement input double; wp1 output double; wp2 output double; wpEnabl input double
function [wp0,wp1, wp2] = getNextWP(wpStart, wpCount, swIncrement, wpEnabl)

% Declare static variables
persistent fromWP;
persistent toWP;
persistent totoWP;

%initialize the static variables
if isempty(fromWP)
    fromWP = uint8(wpStart);
    toWP = uint8(fromWP+1);
    % check if there are more than 2 WPs
    if wpCount > toWP + 1
        totoWP = uint8(toWP+1);
    else
        totoWP = uint8(fromWP);
    end
end

%if WP Nav was just enabled
if wpEnabl == 1
    fromWP = uint8(0);
    toWP = uint8(1);
    totoWP = uint8(2);
end;

% if there is a change of wp
if swIncrement == 1
    fromWP = toWP;
    toWP = totoWP;
    totoWP = totoWP +1;
    if (totoWP>wpCount)
        totoWP = wpStart;
    end
end

wp0 = fromWP;
wp1 = toWP;
wp2 = totoWP;

== matlab function negprotect ==
  data: val input double; zpVal output double
function zpVal = negProt(val)
% This block supports an embeddable subset of the MATLAB language.
% See the help menu for details. 

if val >= single(0.001)
    zpVal = val;
else
    zpVal = single(0.001);
end

== matlab function Navigation/Compute WP Index/Compute Modified L1/Get Circles/Compute Circles ==
  data: sd input double; O output double; cd input double; WP1 input double; R input double; T1 input double; P output double; Pch output double; T2 input double; PchB output double
function [O,P,Pch, PchB] = getO(sd, cd, WP1, R, T1, T2)
    % This block supports an embeddable subset of the MATLAB language.
    % See the help menu for details.

    % rotate the vector delta degrees
    r_vec = zeros(3,1);
    r_vec(1) = -T1(1)*cd -T1(2)*sd;
    r_vec(2) = T1(1)*sd -T1(2)*cd;

    %compute M
    if localAbs(sd)>0.01
        M = localAbs(R/sd);
    else
        M = 0;
    end

    %find the distance from WP
    P = M*cd;

    % find the center of the circle
    O = WP1 + r_vec.*M;

    % find the tangent points
    Pch = WP1-T1*P;
    PchB = WP1 + T2*P;
end

function absVal = localAbs(x)
    if x < 0
        absVal = -1*x;
    else
        absVal = x;
    end
end

== matlab function dsPIC_SQRT/negprotect ==
  data: val input double; zpVal output double
function zpVal = negProt(val)
% This block supports an embeddable subset of the MATLAB language.
% See the help menu for details. 

if val >= single(0.001)
    zpVal = val;
else
    zpVal = single(0.001);
end

== matlab function Navigation/Bank to Psi Dot/negprotect ==
  data: val input double; zpVal output double
function zpVal = negProt(val)
% This block supports an embeddable subset of the MATLAB language.
% See the help menu for details. 

if val >= single(0.001)
    zpVal = val;
else
    zpVal = single(0.001);
end

== matlab function Navigation/Park, Deyst & How Lat Accel Cmd/Compute Eta/negprotect ==
  data: val input double; zpVal output double
function zpVal = negProt(val)
% This block supports an embeddable subset of the MATLAB language.
% See the help menu for details. 

if val >= single(0.001)
    zpVal = val;
else
    zpVal = single(0.001);
end

== matlab function Navigation/Park, Deyst & How Lat Accel Cmd/Compute Eta/negprotect1 ==
  data: val input double; zpVal output double
function zpVal = negProt(val)
% This block supports an embeddable subset of the MATLAB language.
% See the help menu for details. 

if val >= single(0.001)
    zpVal = val;
else
    zpVal = single(0.001);
end

== matlab function Singnal Routing & Conditioning/myMux Fun3 ==
  data: u1 input double; y output double; u2 input double; u3 input double
function y = myMux(u1, u2, u3)
% This block supports an embeddable subset of the MATLAB language.
% See the help menu for details. 

y = [u1(1); u2(1); u3(1)];

== matlab function Singnal Routing & Conditioning/3D LowPass w/Initial Condition/myMux Fun1 ==
  data: u1 input double; y output double; u2 input double; u3 input double
function y = myMux(u1, u2, u3)
% This block supports an embeddable subset of the MATLAB language.
% See the help menu for details. 

y = [u1(1); u2(1); u3(1)];

== matlab function InnerLoop/Longitudinal Channel/0.5 sec  tau for Turns/Embedded MATLAB Function ==
  data: u input double; y output double; T input double; f input double
function y = fcn(u,T,f)
% This block supports an embeddable subset of the MATLAB language.
% See the help menu for details. 

persistent a
persistent b
persistent y_km1
persistent u_km1
if isempty(a)
    %tf = [T*omega/(2+T*omega) T*omega/(2+T*omega)],[1 (T*omega-2)/(T*omega+2)]
    %tf = [a a],[1 -b]
    omega = 2*pi*f;
    a=T*omega/(2+T*omega);
    b=-(T*omega-2)/(T*omega+2);
    y_km1=u;
    u_km1=u;
end

y = a*(u+u_km1)+b*y_km1;
y_km1=y;
u_km1=u;

== matlab function InnerLoop/Longitudinal Channel/Compute Airspeed/Subsystem1/negprotect ==
  data: val input double; zpVal output double
function zpVal = negProt(val)
% This block supports an embeddable subset of the MATLAB language.
% See the help menu for details. 

if val >= single(0.001)
    zpVal = val;
else
    zpVal = single(0.001);
end

== matlab function InnerLoop/Longitudinal Channel/myMux Fun1 ==
  data: u1 input double; y output double; u2 input double; u3 input double
function y = myMux(u1, u2, u3)
% This block supports an embeddable subset of the MATLAB language.
% See the help menu for details. 

y = [u1(1); u2(1); u3(1)];

== matlab function Sensor Blocks/Baro Alt/Baro Altimeter/Enables/Disables the Computation of initial Baro Bias ==
  data: tOut output double
function tOut = getTIni

persistent aveCount;
persistent tIni;

if isempty(aveCount)
    aveCount =1;
    tIni = 1;
end;

if aveCount < 2500
    aveCount = aveCount + 1;
end

if aveCount == 2500
    tIni =0;
    aveCount = aveCount + 1;
end

tOut = tIni;

%if aveCount > 500
%    tIni = 0;
%end

% if isempty(aveCount)
%     aveCount =1;
%     initBias = [0.0 0.0 0.0]';
% end;
%     
% if (aveCount<10)
%     initBias = initBias+ Raw;
%     bias = initBias/aveCount;
%     aveCount = aveCount +1;
% end;
% 
% if (aveCount == 10)
%     initBias = initBias/(aveCount-1);
%     aveCount = 100;
% end;
% 
% if (aveCount == 100)
%     bias = initBias;
% end;

== matlab function Singnal Routing & Conditioning/Ellipse Correction/myMux Fun3 ==
  data: u1 input double; y output double; u2 input double; u3 input double
function y = myMux(u1, u2, u3)
% This block supports an embeddable subset of the MATLAB language.
% See the help menu for details. 

y = [u1(1); u2(1); u3(1)];

== matlab function Control Blocks/Longitudinal Channel/0.5 sec  tau for Turns/Embedded MATLAB Function ==
  data: u input double; y output double; T input double; f input double
function y = fcn(u,T,f)
% This block supports an embeddable subset of the MATLAB language.
% See the help menu for details. 

persistent a
persistent b
persistent y_km1
persistent u_km1
if isempty(a)
    %tf = [T*omega/(2+T*omega) T*omega/(2+T*omega)],[1 (T*omega-2)/(T*omega+2)]
    %tf = [a a],[1 -b]
    omega = 2*pi*f;
    a=T*omega/(2+T*omega);
    b=-(T*omega-2)/(T*omega+2);
    y_km1=u;
    u_km1=u;
end

y = a*(u+u_km1)+b*y_km1;
y_km1=y;
u_km1=u;

== matlab function Control Blocks/Lateral Channel/Sideslip Compensation/Bank to Psi Dot/negprotect ==
  data: val input double; zpVal output double
function zpVal = negProt(val)
% This block supports an embeddable subset of the MATLAB language.
% See the help menu for details. 

if val >= single(0.001)
    zpVal = val;
else
    zpVal = single(0.001);
end

== matlab function Navigation/Navigation/Normal WP Navigation/Embedded MATLAB Function ==
  data: wpEnable input double; reached output double; didReachIP input double
function reached = didUAVReachIp(wpEnable, didReachIP)
% This functions keeps track if the IP has been reached and if so
% it disables homing of IP until WP is reset

persistent persistentDidReachIP;


% initialize the persistent and the return value to 1
% so WP, and not homing, is active by default
if isempty(persistentDidReachIP)
    persistentDidReachIP =  uint8(0);
end


% this is just turned on for one sample 
% inmediatley upon enabling the navigation.
% Reset the flag the the IP was reached
if wpEnable
    persistentDidReachIP = uint8(0);
end

% Once the IP is reached the the persistent variable
% preserves the values until reset
if didReachIP
    persistentDidReachIP = uint8(1);
end;

reached = persistentDidReachIP;

== matlab function Navigation/Navigation/L2+/Get Sin, Cos eta/Get Groundspeed/Zero out Z1 ==
  data: P output double; Pin input double
function P = P2D(Pin)
% This block supports an embeddable subset of the MATLAB language.
% See the help menu for details. 

P = [Pin(1); Pin(2); 0];

== matlab function Navigation/get WP Coord from Index/Get WP from idx SIM/Zero out Z2 ==
  data: y output double; idx input double; vect input double
function y = GetVectorElement(idx , vect)
% This block supports an embeddable subset of the MATLAB language.
% See the help menu for details. 

y = vect(idx);

== matlab function Navigation/get WP Coord from Index/Get WP from idx SIM/Zero out Z1 ==
  data: y output double; idx input double; vect input double
function y = GetVectorElement(idx , vect)
% This block supports an embeddable subset of the MATLAB language.
% See the help menu for details. 

y = vect(idx);

== matlab function Navigation/get WP Coord from Index/Get WP from idx SIM/Zero out Z3 ==
  data: y output double; idx input double; vect input double
function y = GetVectorElement(idx , vect)
% This block supports an embeddable subset of the MATLAB language.
% See the help menu for details. 

y = vect(idx);

== matlab function Navigation/Navigation/myMux Fun6 ==
  data: u1 input double; y output double; u2 input double; u3 input double
function y = myMux(u1, u2, u3)
% This block supports an embeddable subset of the MATLAB language.
% See the help menu for details. 

y = [u1(1); u2(1); u3(1)];

== matlab function Sensor Blocks/Pitot Control End/ 0.3 sec tau for high speeds/Embedded MATLAB Function ==
  data: u input double; y output double; T input double; f input double
function y = fcn(u,T,f)
% This block supports an embeddable subset of the MATLAB language.
% See the help menu for details. 

persistent a
persistent b
persistent y_km1
persistent u_km1
if isempty(a)
    %tf = [T*omega/(2+T*omega) T*omega/(2+T*omega)],[1 (T*omega-2)/(T*omega+2)]
    %tf = [a a],[1 -b]
    omega = 2*pi*f;
    a=T*omega/(2+T*omega);
    b=-(T*omega-2)/(T*omega+2);
    y_km1=u;
    u_km1=u;
end

y = a*(u+u_km1)+b*y_km1;
y_km1=y;
u_km1=u;

== matlab function Sensor Blocks/Baro Alt/Tustin Lowpass, Auto Initial Condition/Embedded MATLAB Function ==
  data: u input double; y output double; T input double; f input double
function y = fcn(u,T,f)
% This block supports an embeddable subset of the MATLAB language.
% See the help menu for details. 

persistent a
persistent b
persistent y_km1
persistent u_km1
if isempty(a)
    %tf = [T*omega/(2+T*omega) T*omega/(2+T*omega)],[1 (T*omega-2)/(T*omega+2)]
    %tf = [a a],[1 -b]
    omega = 2*pi*f;
    a=T*omega/(2+T*omega);
    b=-(T*omega-2)/(T*omega+2);
    y_km1=u;
    u_km1=u;
end

y = a*(u+u_km1)+b*y_km1;
y_km1=y;
u_km1=u;

== matlab function Control Blocks/Lateral Channel/0.016 sec  tau/Embedded MATLAB Function ==
  data: u input double; y output double; T input double; f input double
function y = fcn(u,T,f)
% This block supports an embeddable subset of the MATLAB language.
% See the help menu for details. 

persistent a
persistent b
persistent y_km1
persistent u_km1
if isempty(a)
    %tf = [T*omega/(2+T*omega) T*omega/(2+T*omega)],[1 (T*omega-2)/(T*omega+2)]
    %tf = [a a],[1 -b]
    omega = 2*pi*f;
    a=T*omega/(2+T*omega);
    b=-(T*omega-2)/(T*omega+2);
    y_km1=u;
    u_km1=u;
end

y = a*(u+u_km1)+b*y_km1;
y_km1=y;
u_km1=u;

== matlab function Navigation/Navigation/Normal WP Navigation/computeCurrentWP ==
  data: WPSwitch input double; maxWp input double; IPReached input double; WP0 output double; WP1 output double
function [WP0,WP1] = computeCurrentWP(WPSwitch, maxWp, IPReached)
% This functions keeps track if the IP has been reached and if so
% it disables homing of IP until WP is reset

persistent fromWp;
persistent toWp;

% initialize the persistent and the return value to 1
% so WP, and not homing, is active by default
if isempty(fromWp)
    fromWp =  uint8(1);
    toWp = uint8(2);
end

if WPSwitch
    fromWp = toWp;
    toWp = toWp +1;
    if (toWp > maxWp)
        toWp = uint8(1);
    end
end


% this is jturned on long as we have not reached IP 
if ~IPReached
    fromWp = uint8(1);
    toWp = uint8(2);
end



WP0 = fromWp;
WP1 = toWp;

== matlab function Navigation/Navigation/Normal WP Navigation/Get Frenet/Zero out Z1 ==
  data: P output double; Pin input double
function P = P2D(Pin)
% This block supports an embeddable subset of the MATLAB language.
% See the help menu for details. 

P = [Pin(1); Pin(2); 0];

== matlab function Navigation/Navigation/Normal WP Navigation/Get Frenet/Zero out Z2 ==
  data: P output double; Pin input double
function P = P2D(Pin)
% This block supports an embeddable subset of the MATLAB language.
% See the help menu for details. 

P = [Pin(1); Pin(2); 0];

== matlab function InnerLoop/Longitudinal Channel/ 0.3 sec tau for high speeds/Embedded MATLAB Function ==
  data: u input double; y output double; T input double; f input double
function y = fcn(u,T,f)
% This block supports an embeddable subset of the MATLAB language.
% See the help menu for details. 

persistent a
persistent b
persistent y_km1
persistent u_km1
if isempty(a)
    %tf = [T*omega/(2+T*omega) T*omega/(2+T*omega)],[1 (T*omega-2)/(T*omega+2)]
    %tf = [a a],[1 -b]
    omega = 2*pi*f;
    a=T*omega/(2+T*omega);
    b=-(T*omega-2)/(T*omega+2);
    y_km1=u;
    u_km1=u;
end

y = a*(u+u_km1)+b*y_km1;
y_km1=y;
u_km1=u;

== matlab function Navigation/Navigation/L2+/Get Sin, Cos eta/negprotect ==
  data: val input double; zpVal output double
function zpVal = negProt(val)
% This block supports an embeddable subset of the MATLAB language.
% See the help menu for details. 

if val >= single(0.0001)
    zpVal = val;
else
    zpVal = single(0.0001);
end

== matlab function Navigation/Navigation/L2+/L2+/negprotect ==
  data: val input double; zpVal output double
function zpVal = negProt(val)
% This block supports an embeddable subset of the MATLAB language.
% See the help menu for details. 

if val >= single(0.0001)
    zpVal = val;
else
    zpVal = single(0.0001);
end

== matlab function Navigation/Navigation/Normal WP Navigation/Get Frenet/Zero out Z3 ==
  data: P output double; Pin input double
function P = P2D(Pin)
% This block supports an embeddable subset of the MATLAB language.
% See the help menu for details. 

P = [Pin(1); Pin(2); 0];

== matlab function Navigation/Navigation/Normal WP Navigation/Zero out Z2 ==
  data: P output double; Pin input double
function P = P2D(Pin)
% This block supports an embeddable subset of the MATLAB language.
% See the help menu for details. 

P = [Pin(1); Pin(2); 0];
